simulink model "dynamics"  (R2018b)
settings: Solver=VariableStepAuto  StartTime=0.0  StopTime=10  RelTol=1e-3
settings Model: Creator=Srikar  LastModifiedBy=holyCow
settings SFSimCC: SimUseLocalCustomCode=off
settings RTWCC: RTWUseLocalCustomCode=off

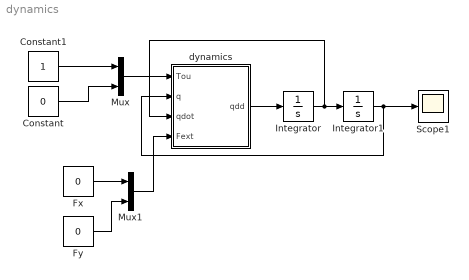
== system dynamics ==
  " Fy " : Constant  Value=0
  Constant : Constant  Value=0
  Constant1 : Constant
  Fx : Constant  Value=0
  Integrator : Integrator
  Integrator1 : Integrator
  Mux : Mux  Inputs=2
  Mux1 : Mux  Inputs=2
  Scope1 : Scope
  dynamics : MATLAB Function  TreatAsAtomicUnit=on
  wires:
  Constant/1 -> Mux/2
  Fx/1 -> Mux1/1
  dynamics/1(qdd) -> Integrator/1
  Constant1/1 -> Mux/1
  " Fy "/1 -> Mux1/2
  Mux1/1 -> dynamics/4(Fext)
  Mux/1 -> dynamics/1(Tou)
  Integrator1/1 -> dynamics/2(q), Scope1/1
  Integrator/1 -> dynamics/3(qdot), Integrator1/1

== matlab function dynamics/dynamics ==
  data: Tou input; qdd output; q input; qdot input; Fext input
function qdd   = fcn(Tou, q, qdot, Fext)
b = 0.265; %body
a = 0.170; %arm
g = 9.81;

mBody = 2; %body
mArm = 0.1; %arm

q1 = q(1);
q2 = q(2);

m11 = mBody*b^2 + mArm*(b^2 + 2*b*a*cos(q2)+a^2);
m12 = mArm*(b*a*cos(q2) + a^2);
m21 = mArm*(b*a*cos(q2) + a^2);
m22 = mArm*a^2;

M = [m11 m12; m21 m22];

q1d = qdot(1);
q2d = qdot(2);

c11 = -mArm*b*a*sin(q2)*(2*q1d*q2d + q2^2);
c21 = mArm*b*a*q1d^2*sin(q2);

Cqdot = [c11; c21];

g11 = (mBody + mArm)*b*g*cos(q1) + mArm*g*a*cos(q1 + q2);
g21 = mArm*g*a*cos(q1 + q2);

G = [g11; g21];

j11 = -b*sin(q1) - a*sin(q1 + q2);
j12 = -a*sin(q1 + q2);
j21 = b*cos(q1) + a*cos(q1 + q2);
j22 = a*cos(q1 + q2);

J = [j11 j12; j21 j22];

Minv=inv(M);
qdd = Minv * (Tou - Cqdot - G - J'*Fext);
